simulink model "MSDR_and_BOP_v1_1"  (R2019a)
settings: Solver=ode45  StartTime=0.0  StopTime=15000  FixedStep=0.1  MaxStep=10
values from neighbouring files (symbols this model uses):
  a_f = -3.22E-5    (= -3.22e-05)    [MSDR_parameters_v1_1.m]
  a_g = +2.35E-5    (= 2.35e-05)    [MSDR_parameters_v1_1.m]
  A_s = 1.2245    [MSDR_parameters_v1_1.m]
  beta = [0.000223, 0.001457, 0.001307, 0.002628, 0.000766, 0.000280]    [MSDR_parameters_v1_1.m]
  beta_t = sum(beta)    [MSDR_parameters_v1_1.m]
  ce1 = 1.2471e-07    [MSDR_parameters_v1_1.m]
  ce2 = 5.3816e-14    [MSDR_parameters_v1_1.m]
  ce3 = 3.3721e-08    [MSDR_parameters_v1_1.m]
  Cp_fw = 3200.448e-6    (= 0.003200448)    [MSDR_parameters_v1_1.m]
  Cp_hr = 0.0021520    (= 0.002152)    [MSDR_parameters_v1_1.m]
  Cp_p = Cp_s_shx    (= 0.00154912)    [MSDR_parameters_v1_1.m]
  Cp_s = Cp_s*1e-6    (= 3.588208e-09)    [MSDR_parameters_v1_1.m]
  Cp_s_shx = 1549.12e-6    (= 0.00154912)    [MSDR_parameters_v1_1.m]
  Cp_sc = 4761.392e-6    (= 0.004761392)    [MSDR_parameters_v1_1.m]
  Cp_w = 456.056e-6    (= 0.000456056)    [MSDR_parameters_v1_1.m]
  D_it = 0.0141478    [MSDR_parameters_v1_1.m]
  D_ot = 0.015875    [MSDR_parameters_v1_1.m]
  dHs_dPs = -0.042433622114357    (= -0.0424336221144)    [MSDR_parameters_v1_1.m]
  eta_hp_isen = 0.861    [MSDR_parameters_v1_1.m]
  eta_lp_isen = 0.861    [MSDR_parameters_v1_1.m]
  gamma_I = 5.1135e-2    (= 0.051135)    [MSDR_parameters_v1_1.m]
  gamma_Xe = 1.1628e-2    (= 0.011628)    [MSDR_parameters_v1_1.m]
  H_fwh1 = 0.46009    [MSDR_parameters_v1_1.m]
  h_fwh1 = 0.5927    [MSDR_parameters_v1_1.m]
  H_fwh2 = 0.6784    [MSDR_parameters_v1_1.m]
  h_fwh2 = 0.5927    [MSDR_parameters_v1_1.m]
  H_lp_isen = 958.4*1054.35e-6/0.45359237    (= 2.22774699671)    [MSDR_parameters_v1_1.m]
  H_nc = 3.2952    [MSDR_parameters_v1_1.m]
  h_pw = h_s_shx    (= 0.00567446)    [MSDR_parameters_v1_1.m]
  H_rh = 2.8115    [MSDR_parameters_v1_1.m]
  h_wb = 13349.334646671E-6    (= 0.0133493346467)    [MSDR_parameters_v1_1.m]
  h_ws = 5732.378387768E-6    (= 0.00573237838777)    [MSDR_parameters_v1_1.m]
  h_wsc = 8385.005556375E-6    (= 0.00838500555638)    [MSDR_parameters_v1_1.m]
  hA_fg = [h_fg*A_fg/2, h_fg*A_fg/2]    [MSDR_parameters_v1_1.m]
  hA_p_phx1 = h_p_phx*A_p_phx    [MSDR_parameters_v1_1.m]
  hA_p_phx2 = h_p_phx*A_p_phx    [MSDR_parameters_v1_1.m]
  hA_p_phx3 = h_p_phx*A_p_phx    [MSDR_parameters_v1_1.m]
  hA_p_phx4 = h_p_phx*A_p_phx    [MSDR_parameters_v1_1.m]
  hA_p_phx5 = h_p_phx*A_p_phx    [MSDR_parameters_v1_1.m]
  hA_p_phx6 = h_p_phx*A_p_phx    [MSDR_parameters_v1_1.m]
  hA_p_shx1 = h_p_shx*A_p_shx    [MSDR_parameters_v1_1.m]
  hA_p_shx2 = h_p_shx*A_p_shx    [MSDR_parameters_v1_1.m]
  hA_p_shx3 = h_p_shx*A_p_shx    [MSDR_parameters_v1_1.m]
  hA_p_shx4 = h_p_shx*A_p_shx    [MSDR_parameters_v1_1.m]
  hA_p_shx5 = h_p_shx*A_p_shx    [MSDR_parameters_v1_1.m]
  hA_p_shx6 = h_p_shx*A_p_shx    [MSDR_parameters_v1_1.m]
  hA_s_phx1 = h_s_phx*A_s_phx    [MSDR_parameters_v1_1.m]
  hA_s_phx2 = h_s_phx*A_s_phx    [MSDR_parameters_v1_1.m]
  hA_s_phx3 = h_s_phx*A_s_phx    [MSDR_parameters_v1_1.m]
  hA_s_phx4 = h_s_phx*A_s_phx    [MSDR_parameters_v1_1.m]
  hA_s_phx5 = h_s_phx*A_s_phx    [MSDR_parameters_v1_1.m]
  hA_s_phx6 = h_s_phx*A_s_phx    [MSDR_parameters_v1_1.m]
  hA_s_shx1 = h_s_shx*A_s_shx    [MSDR_parameters_v1_1.m]
  hA_s_shx2 = h_s_shx*A_s_shx    [MSDR_parameters_v1_1.m]
  hA_s_shx3 = h_s_shx*A_s_shx    [MSDR_parameters_v1_1.m]
  hA_s_shx4 = h_s_shx*A_s_shx    [MSDR_parameters_v1_1.m]
  hA_s_shx5 = h_s_shx*A_s_shx    [MSDR_parameters_v1_1.m]
  hA_s_shx6 = h_s_shx*A_s_shx    [MSDR_parameters_v1_1.m]
  I_0 = gamma_I*Sig_f_msdr*phi_0/lam_I    (= 4.38204721773e+16)    [MSDR_parameters_v1_1.m]
  Ifa = [0.25, 0.25]    [MSDR_parameters_v1_1.m]
  Ifb = [0.25, 0.25]    [MSDR_parameters_v1_1.m]
  Ig = [0.5, 0.5]    [MSDR_parameters_v1_1.m]
  K_1 = 11.632248097704855    (= 11.6322480977)    [MSDR_parameters_v1_1.m]
  K_4 = b(1)    [MSDR_parameters_v1_1.m]
  K_5 = a(1)    [MSDR_parameters_v1_1.m]
  K_b = 12.834854076292217    (= 12.8348540763)    [MSDR_parameters_v1_1.m]
  K_b_hp = 0.1634    [MSDR_parameters_v1_1.m]
  K_b_lp = 0.2174    [MSDR_parameters_v1_1.m]
  K_sc = -17.615718797133468    (= -17.6157187971)    [MSDR_parameters_v1_1.m]
  ka = [0.235, 0.235]    [MSDR_parameters_v1_1.m]
  kb = [0.235, 0.235]    [MSDR_parameters_v1_1.m]
  kga = [0.015, 0.015]    [MSDR_parameters_v1_1.m]
  kgb = [0.015, 0.015]    [MSDR_parameters_v1_1.m]
  L = 8.5344    [MSDR_parameters_v1_1.m]
  L_b = 2.3645    [MSDR_parameters_v1_1.m]
  L_s = 4.723    [MSDR_parameters_v1_1.m]
  Lam = 2.400E-04    (= 0.00024)    [MSDR_parameters_v1_1.m]
  lam = [0.0124, 0.0305, 0.111, 0.301, 1.14, 3.01]    [MSDR_parameters_v1_1.m]
  lam_bubl = 2.0e-2    (= 0.02)    [MSDR_parameters_v1_1.m]
  lam_I = 2.875e-5    (= 2.875e-05)    [MSDR_parameters_v1_1.m]
  lam_Xe = 2.0916e-5    (= 2.0916e-05)    [MSDR_parameters_v1_1.m]
  m_3m = W_3*2    (= 8618.207327)    [MSDR_parameters_v1_1.m]
  m_fm = W_f*2    (= 9978.96)    [MSDR_parameters_v1_1.m]
  m_sb = 1717    [MSDR_parameters_v1_1.m]
  M_stm = 0.018    [MSDR_parameters_v1_1.m]
  mb_cpb = 2.689619410657651e+00    (= 2.68961941066)    [MSDR_parameters_v1_1.m]
  mcp_fa = mfa*Cp_f    [MSDR_parameters_v1_1.m]
  mcp_fb = mfb*Cp_f    [MSDR_parameters_v1_1.m]
  mcp_g = mg*Cp_g    [MSDR_parameters_v1_1.m]
  mcp_p_phx1 = Cp_p_phx*mp_phx1    [MSDR_parameters_v1_1.m]
  mcp_p_phx2 = Cp_p_phx*mp_phx2    [MSDR_parameters_v1_1.m]
  mcp_p_phx3 = Cp_p_phx*mp_phx3    [MSDR_parameters_v1_1.m]
  mcp_p_phx4 = Cp_p_phx*mp_phx4    [MSDR_parameters_v1_1.m]
  mcp_p_phx5 = Cp_p_phx*mp_phx5    [MSDR_parameters_v1_1.m]
  mcp_p_phx6 = Cp_p_phx*mp_phx6    [MSDR_parameters_v1_1.m]
  mcp_p_shx1 = Cp_p_shx*mp_shx1    [MSDR_parameters_v1_1.m]
  mcp_p_shx2 = Cp_p_shx*mp_shx2    [MSDR_parameters_v1_1.m]
  mcp_p_shx3 = Cp_p_shx*mp_shx3    [MSDR_parameters_v1_1.m]
  mcp_p_shx4 = Cp_p_shx*mp_shx4    [MSDR_parameters_v1_1.m]
  mcp_p_shx5 = Cp_p_shx*mp_shx5    [MSDR_parameters_v1_1.m]
  mcp_p_shx6 = Cp_p_shx*mp_shx6    [MSDR_parameters_v1_1.m]
  mcp_s_phx1 = Cp_s_phx*ms_phx1    [MSDR_parameters_v1_1.m]
  mcp_s_phx2 = Cp_s_phx*ms_phx2    [MSDR_parameters_v1_1.m]
  mcp_s_phx3 = Cp_s_phx*ms_phx3    [MSDR_parameters_v1_1.m]
  mcp_s_phx4 = Cp_s_phx*ms_phx4    [MSDR_parameters_v1_1.m]
  mcp_s_phx5 = Cp_s_phx*ms_phx5    [MSDR_parameters_v1_1.m]
  mcp_s_phx6 = Cp_s_phx*ms_phx6    [MSDR_parameters_v1_1.m]
  mcp_s_shx1 = Cp_s_shx*ms_shx1    [MSDR_parameters_v1_1.m]
  mcp_s_shx2 = Cp_s_shx*ms_shx1    [MSDR_parameters_v1_1.m]
  mcp_s_shx3 = Cp_s_shx*ms_shx1    [MSDR_parameters_v1_1.m]
  mcp_s_shx4 = Cp_s_shx*ms_shx1    [MSDR_parameters_v1_1.m]
  mcp_s_shx5 = Cp_s_shx*ms_shx1    [MSDR_parameters_v1_1.m]
  mcp_s_shx6 = Cp_s_shx*ms_shx1    [MSDR_parameters_v1_1.m]
  mcp_t_phx1 = Cp_t_phx*mt_phx1    [MSDR_parameters_v1_1.m]
  mcp_t_phx2 = Cp_t_phx*mt_phx2    [MSDR_parameters_v1_1.m]
  mcp_t_phx3 = Cp_t_phx*mt_phx3    [MSDR_parameters_v1_1.m]
  mcp_t_phx4 = Cp_t_phx*mt_phx4    [MSDR_parameters_v1_1.m]
  mcp_t_phx5 = Cp_t_phx*mt_phx5    [MSDR_parameters_v1_1.m]
  mcp_t_phx6 = Cp_t_phx*mt_phx6    [MSDR_parameters_v1_1.m]
  mcp_t_shx1 = Cp_t_phx*mt_shx1    [MSDR_parameters_v1_1.m]
  ... (+177 more)
undefined symbols (not defined in the file or in its folder): C0, H_con_table, H_convap_table, H_rh_table, H_rh_table1, H_rh_table2, H_rhvap_table, H_s_table, H_table, hA_p_thx1, hA_p_thx2, hA_p_thx3, hA_s_thx1, hA_s_thx2, hA_s_thx3, ln, mcp_p_thx1, mcp_p_thx2, mcp_p_thx3, mcp_s_thx1, mcp_s_thx2, mcp_s_thx3, mcp_t_thx1, mcp_t_thx2, mcp_t_thx3, mp_thx1, mp_thx2, mp_thx3, ms_thx1, ms_thx2, ms_thx3, P_con_table, P_nc_table, P_rh_table, P_rh_table1, pres_table, rho_rh_table, rho_table, SV_nc_table, T0_p_thx1, T0_p_thx2, T0_p_thx3, T0_s_thx1, T0_s_thx2, T0_s_thx3, T0_t_thx1, T0_t_thx2, T0_t_thx3, temp_table, u14, Wp_thx1, Wp_thx2, Wp_thx3, Ws_thx1, Ws_thx2, Ws_thx3
libraries: simulink x10
(part 2 of 4)

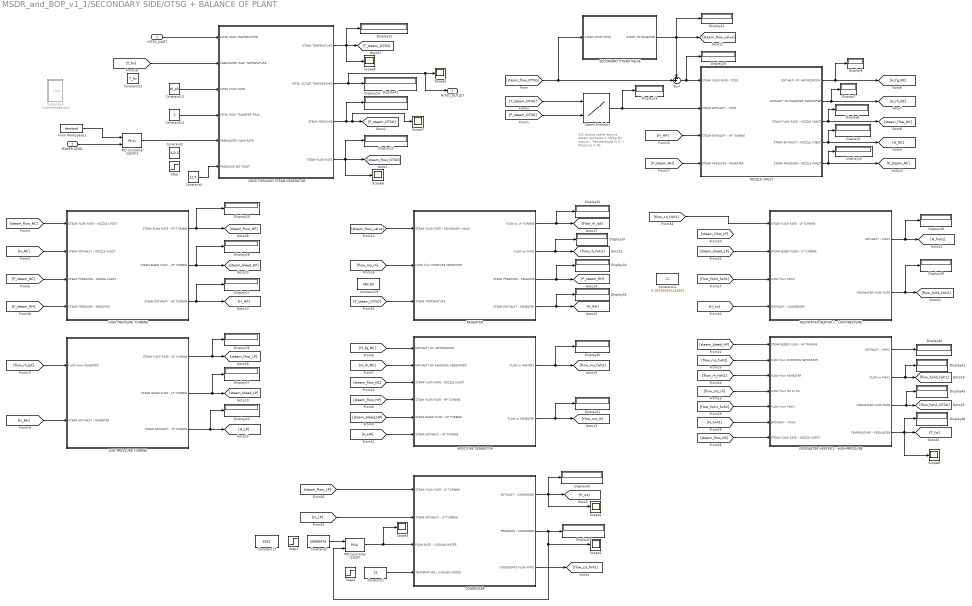
== system MSDR_and_BOP_v1_1/SECONDARY SIDE/OTSG + BALANCE OF PLANT ==
  note: 2-D lookup table returns steam enthalpy in MJ/kg for inputs i. Temperature in C, ii. Pressure in Pa
  HITEC_INLET : Inport
  POWER LEVEL : Inport  Port=2
  CONDENSER : Subsystem
  Constant1 : Constant  Value=15
  Constant11 : Constant  Value=0.160386626432892
  Constant12 : Constant  Value=T_fw
  Constant13 : Constant  Value=W_p0
  Constant14 : Constant
  Constant17 : Constant  Value=2552
  Constant19 : Constant  Value=482.63
  Constant2 : Constant  Value=322.5
  Constant3 : Constant  Value=.00689476
  Constant4 : Constant  Value=12.5
  Display{6..15,26..47} (32 alike) : Display
  FEEDWATER HEATER 1 - LOW-PRESSURE : Subsystem
  FEEDWATER HEATER 2 - HIGH-PRESSURE : Subsystem
  From Workspace1 : FromWorkspace  VariableName=demand  SampleTime=1  Interpolate=off  OutputAfterFinalValue=Holding final value
  HIGH PRESSURE TURBINE : Subsystem
  LOW PRESSURE TURBINE : Subsystem
  MOISTURE SEPARATOR : Subsystem
  NOZZLE CHEST : Subsystem
  ONCE-THROUGH STEAM GENERATOR : Subsystem
  PID Controller (2DOF) : simulink/Continuous/PID Controller (2DOF)  Controller=PI  Form=Ideal  TimeDomain=Continuous-time  SampleTime=-1  IntegratorMethod=Forward Euler  FilterMethod=Forward Euler  ControllerParametersSource=internal  P=-10020.0301151595  I=2.45363177832513  D=1  UseFilter=on  N=100  b=8.59224632013355e-05  c=1  TunerSelectOption=Transfer Function Based (PID Tuner App)  InitialConditionSource=internal  InitialConditionForIntegrator=0  InitialConditionForFilter=0  DifferentiatorICPrevScaledInput=0  ExternalReset=none  TrackingMode=off  Kt=1  LimitOutput=on  UpperSaturationLimit=100000  LowerSaturationLimit=10  LinearizeAsGain=off  AntiWindupMode=none  Kb=1  POutMin=[]  POutMax=[]  IOutMin=[]  IOutMax=[]  DOutMin=[]  DOutMax=[]  NOutMin=[]  NOutMax=[]  bOutMin=[]  bOutMax=[]  cOutMin=[]  cOutMax=[]  SumOutMin=[]  SumOutMax=[]  SaturationOutMin=[]  SaturationOutMax=[]  PParamMin=[]  PParamMax=[]  IParamMin=[]  IParamMax=[]  DParamMin=[]  DParamMax=[]  NParamMin=[]  NParamMax=[]  bParamMin=[]  bParamMax=[]  cParamMin=[]  cParamMax=[]  KbParamMin=[]  KbParamMax=[]  KtParamMin=[]  KtParamMax=[]  KbOutMin=[]  KbOutMax=[]  KtOutMin=[]  KtOutMax=[]  IntegratorOutMin=[]  IntegratorOutMax=[]  FilterOutMin=[]  FilterOutMax=[]  SumI1OutMin=[]  SumI1OutMax=[]  SumI2OutMin=[]  SumI2OutMax=[]  SumI3OutMin=[]  SumI3OutMax=[]  SumI4OutMin=[]  SumI4OutMax=[]  SumDOutMin=[]  SumDOutMax=[]  Sum1OutMin=[]  Sum1OutMax=[]  Sum2OutMin=[]  Sum2OutMax=[]  Sum3OutMin=[]  Sum3OutMax=[]  DifferentiatorOutMin=[]  DifferentiatorOutMax=[]  FilterDiffOutCoefMin=[]  FilterDiffOutCoefMax=[]  ReciprocalOutMin=[]  ReciprocalOutMax=[]  SumDenOutMin=[]  SumDenOutMax=[]  SumNumOutMin=[]  SumNumOutMax=[]  DivideOutMin=[]  DivideOutMax=[]  IntegratorContinuousStateAttributes=''  IntegratorStateMustResolveToSignalObject=off  IntegratorRTWStateStorageClass=Auto  FilterContinuousStateAttributes=''  FilterStateMustResolveToSignalObject=off  FilterRTWStateStorageClass=Auto  ParallelPVariant=Passthrough  IdealPVariant=InternalParameters  IVariant=InternalParameters  DVariant=Disabled  bVariant=InternalParameters  cVariant=Disabled  IntegratorVariant=Continuous  SatVariant=Enabled  AWVariant=Passthrough  PCopyVariant=Disabled  TRVariant=Disabled  FdbkBlocksVariant=Forward  IdealPFdbkVariant=Disabled  SatFdbkVariant=Disabled  DerivativeFilterVariant=Disabled  NVariant=Disabled  NCopyVariant=Disabled_SignalSpec  FilterICVariant=Disabled  IntegratorICVariant=InternalICs  ExternalResetVariant=Disabled  TRSumVariant=Passthrough  SumFdbkVariant=Disabled  SumVariant=Sum_PI
  PID Controller (2DOF)1 : simulink/Continuous/PID Controller (2DOF)  Controller=PI  Form=Parallel  TimeDomain=Continuous-time  SampleTime=-1  IntegratorMethod=Forward Euler  FilterMethod=Forward Euler  ControllerParametersSource=internal  P=250  I=5  D=1  UseFilter=on  N=100  b=1  c=1  TunerSelectOption=Transfer Function Based (PID Tuner App)  InitialConditionSource=internal  InitialConditionForIntegrator=0  InitialConditionForFilter=0  DifferentiatorICPrevScaledInput=0  ExternalReset=none  TrackingMode=off  Kt=1  LimitOutput=on  UpperSaturationLimit=1000000  LowerSaturationLimit=1  LinearizeAsGain=on  AntiWindupMode=none  Kb=1  POutMin=[]  POutMax=[]  IOutMin=[]  IOutMax=[]  DOutMin=[]  DOutMax=[]  NOutMin=[]  NOutMax=[]  bOutMin=[]  bOutMax=[]  cOutMin=[]  cOutMax=[]  SumOutMin=[]  SumOutMax=[]  SaturationOutMin=[]  SaturationOutMax=[]  PParamMin=[]  PParamMax=[]  IParamMin=[]  IParamMax=[]  DParamMin=[]  DParamMax=[]  NParamMin=[]  NParamMax=[]  bParamMin=[]  bParamMax=[]  cParamMin=[]  cParamMax=[]  KbParamMin=[]  KbParamMax=[]  KtParamMin=[]  KtParamMax=[]  KbOutMin=[]  KbOutMax=[]  KtOutMin=[]  KtOutMax=[]  IntegratorOutMin=[]  IntegratorOutMax=[]  FilterOutMin=[]  FilterOutMax=[]  SumI1OutMin=[]  SumI1OutMax=[]  SumI2OutMin=[]  SumI2OutMax=[]  SumI3OutMin=[]  SumI3OutMax=[]  SumI4OutMin=[]  SumI4OutMax=[]  SumDOutMin=[]  SumDOutMax=[]  Sum1OutMin=[]  Sum1OutMax=[]  Sum2OutMin=[]  Sum2OutMax=[]  Sum3OutMin=[]  Sum3OutMax=[]  DifferentiatorOutMin=[]  DifferentiatorOutMax=[]  FilterDiffOutCoefMin=[]  FilterDiffOutCoefMax=[]  ReciprocalOutMin=[]  ReciprocalOutMax=[]  SumDenOutMin=[]  SumDenOutMax=[]  SumNumOutMin=[]  SumNumOutMax=[]  DivideOutMin=[]  DivideOutMax=[]  IntegratorContinuousStateAttributes=''  IntegratorStateMustResolveToSignalObject=off  IntegratorRTWStateStorageClass=Auto  FilterContinuousStateAttributes=''  FilterStateMustResolveToSignalObject=off  FilterRTWStateStorageClass=Auto  ParallelPVariant=InternalParameters  IdealPVariant=Disabled  IVariant=InternalParameters  DVariant=Disabled  bVariant=InternalParameters  cVariant=Disabled  IntegratorVariant=Continuous  SatVariant=Enabled  AWVariant=Passthrough  PCopyVariant=Disabled  TRVariant=Disabled  FdbkBlocksVariant=Forward  IdealPFdbkVariant=Disabled  SatFdbkVariant=Disabled  DerivativeFilterVariant=Disabled  NVariant=Disabled  NCopyVariant=Disabled_SignalSpec  FilterICVariant=Disabled  IntegratorICVariant=InternalICs  ExternalResetVariant=Disabled  TRSumVariant=Passthrough  SumFdbkVariant=Disabled  SumVariant=Sum_PI
  REHEATER : Subsystem
  SECONDARY STEAM VALVE : Subsystem
  Scope{1..8} (8 alike) : Scope
  Steam Enthalpy : Lookup_n-D  BreakpointsForDimension1=temp_table  BreakpointsForDimension2=pres_table  Table=H_s_table  DiagnosticForOutOfRangeInput=Warning  InternalRulePriority=Speed  RndMeth=Simplest  InputSameDT=on
  Step : Step  Time=1000  Before=12.5  After=12  SampleTime=0
  Step1 : Step  Time=1000  Before=0.00689476  After=.00589476  SampleTime=0
  Step2 : Step  Time=1000  Before=25  After=15  SampleTime=0
  Subsystem : Subsystem  Commented=on
  Sum : Sum  Inputs=-+|
  HITEC_OUTLET : Outport
  wires:
  REHEATER/1("FLOW to LP TURBINE ") -> [flow_rh_lpt], Display32/1
  [steam_flow_NC] -> HIGH PRESSURE TURBINE/1(STEAM FLOW RATE - NOZZLE CHEST)
  [steam_bleed_HP] -> MOISTURE SEPARATOR/5(STEAM BLEED FLOW - HP TURBINE)
  [steam_flow_NC] -> MOISTURE SEPARATOR/3(STEAM FLOW RATE - NOZZLE CHEST)
  NOZZLE CHEST/3(STEAM FLOW RATE - NOZZLE CHEST) -> [steam_flow_NC], Display8/1
  [H_rh_NC] -> MOISTURE SEPARATOR/2(ENTHALPY OF REHEATER FEEDWATER)
  NOZZLE CHEST/2(ENTHALPY OF REHEATER FEEDWATER) -> [H_rh_NC], Display7/1
  [H_NC] -> HIGH PRESSURE TURBINE/2(STEAM ENTHALPY - NOZZLE CHEST)
  Steam Enthalpy/1 -> NOZZLE CHEST/2(STEAM ENTHALPY - OTSG), Display13/1
  [steam_flow_HP] -> MOISTURE SEPARATOR/4(STEAM FLOW RATE - HP TURBINE)
  Sum/1 -> Display26/1, NOZZLE CHEST/1(STEAM FLOW RATE - OTSG)
  NOZZLE CHEST/5(STEAM PRESSURE - NOZZLE CHEST) -> [P_steam_NC], Display10/1
  [H_fwh1] -> FEEDWATER HEATER 2 - HIGH-PRESSURE/6(ENTHALPY - FWH1)
  REHEATER/2(FLOW to FWH2) -> [flow_rh_fwh2], Display33/1
  FEEDWATER HEATER 1 - LOW-PRESSURE/1(ENTHALPY - FWH1) -> [H_fwh1], Display38/1
  [flow_rh_fwh2] -> FEEDWATER HEATER 2 - HIGH-PRESSURE/3(FLOW from REHEATER)
  [flow_ms_rh] -> FEEDWATER HEATER 2 - HIGH-PRESSURE/4(FLOW from MS to RH)
  FEEDWATER HEATER 2 - HIGH-PRESSURE/2(FLOW to FWH1) -> Display41/1, [flow_fwh2_fwh1]
  [flow_ms_fwh2] -> FEEDWATER HEATER 2 - HIGH-PRESSURE/2(FLOW from MOISTURE SEPARATOR)
  MOISTURE SEPARATOR/1(FLOW to HEATER2) -> [flow_ms_fwh2], Display30/1
  [flow_fwh2_fwh1] -> FEEDWATER HEATER 1 - LOW-PRESSURE/3(FLOW from FWH2)
  [flow_ms_rh] -> REHEATER/2(FLOW from MOISTURE SEPARATOR)
  MOISTURE SEPARATOR/2(FLOW to REHEATER) -> [flow_ms_rh], Display31/1
  REHEATER/3(STEAM PRESSURE - REHEATER) -> [P_steam_RH], Display34/1
  FEEDWATER HEATER 2 - HIGH-PRESSURE/3(FEEDWATER FLOW RATE) -> Display45/1, [flow_fwh2_OTSG]
  LOW PRESSURE TURBINE/3(STEAM ENTHALPY - LP TURBINE) -> Display42/1, [H_LP]
  [P_steam_NC] -> HIGH PRESSURE TURBINE/3(STEAM PRESSURE - NOZZLE CHEST)
  FEEDWATER HEATER 2 - HIGH-PRESSURE/4(TEMPERATURE - FEEDWATER) -> [T_fw], Scope8/1, Display46/1
  NOZZLE CHEST/4(STEAM ENTHALPY - NOZZLE CHEST) -> [H_NC], Display9/1
  [flow_rh_lpt] -> LOW PRESSURE TURBINE/1(FLOW from REHEATER)
  HIGH PRESSURE TURBINE/3(STEAM ENTHALPY - HP TURBINE) -> [H_HP], Display27/1
  [H_fg_NC] -> MOISTURE SEPARATOR/1(ENTHALPY OF VAPORIZATION)
  [flow_fwh1_fwh2] -> FEEDWATER HEATER 2 - HIGH-PRESSURE/5(FLOW from FWH1)
  [steam_flow_valve] -> REHEATER/1(STEAM FLOW RATE - SECONDARY VALVE)
  ONCE-THROUGH STEAM GENERATOR/4(STEAM FLOW RATE) -> Scope6/1, [steam_flow_OTSG], Display15/1
  [P_steam_OTSG] -> Steam Enthalpy/2
  [H_HP] -> MOISTURE SEPARATOR/6(STEAM ENTHALPY - HP TURBINE)
  SECONDARY STEAM VALVE/1(STEAM TO REHEATER) -> Display11/1, [steam_flow_valve], Sum/1
  [H_HP] -> NOZZLE CHEST/3(STEAM ENTHALPY - HP TURBINE)
  ONCE-THROUGH STEAM GENERATOR/2(HITEC OUTLET TEMPERATURE) -> HITEC_OUTLET/1, Scope5/1, Display47/1
  NOZZLE CHEST/1(ENTHALPY OF VAPORIZATION) -> [H_fg_NC], Display6/1
  [P_steam_RH] -> NOZZLE CHEST/4(STEAM PRESSURE - REHEATER)
  REHEATER/4(STEAM ENTHALPY - REHEATER) -> [H_RH], Display35/1
  LOW PRESSURE TURBINE/2(STEAM BLEED FLOW - LP TURBINE) -> [steam_bleed_LP], Display37/1
  Constant13/1 -> ONCE-THROUGH STEAM GENERATOR/3(HITEC FLOW RATE)
  FEEDWATER HEATER 2 - HIGH-PRESSURE/1(ENTHALPY - FWH2) -> Display40/1
  HIGH PRESSURE TURBINE/1(STEAM FLOW RATE - HP TURBINE) -> [steam_flow_HP], Display29/1
  [T_steam_OTSG] -> REHEATER/3(STEAM TEMPERATURE)
  ONCE-THROUGH STEAM GENERATOR/1(STEAM TEMPERATURE) -> Scope4/1, Display12/1, [T_steam_OTSG]
  Constant14/1 -> ONCE-THROUGH STEAM GENERATOR/4(HITEC HEAT TRANSFER FRAC)
  [T_fw] -> ONCE-THROUGH STEAM GENERATOR/2(FEEDWATER INLET TEMPERATURE)
  [steam_bleed_LP] -> FEEDWATER HEATER 1 - LOW-PRESSURE/2(STEAM BLEED FLOW - LP TURBINE)
  [H_RH] -> LOW PRESSURE TURBINE/2(STEAM ENTHALPY - REHEATER)
  [steam_bleed_HP] -> FEEDWATER HEATER 2 - HIGH-PRESSURE/1(STEAM BLEED FLOW - HP TURBINE)
  ONCE-THROUGH STEAM GENERATOR/3(STEAM PRESSURE) -> Scope7/1, [P_steam_OTSG], Display14/1
  LOW PRESSURE TURBINE/1(STEAM FLOW RATE - LP TURBINE) -> [steam_flow_LP], Display36/1
  [T_steam_OTSG] -> Steam Enthalpy/1
  [P_steam_RH] -> HIGH PRESSURE TURBINE/4(STEAM PRESSURE - REHEATER)
  HIGH PRESSURE TURBINE/2(STEAM BLEED FLOW - HP TURBINE) -> [steam_bleed_HP], Display28/1
  [steam_flow_NC] -> FEEDWATER HEATER 2 - HIGH-PRESSURE/7(STEAM FLOW RATE - NOZZLE CHEST)
  FEEDWATER HEATER 1 - LOW-PRESSURE/2(FEEDWATER FLOW RATE) -> Display39/1, [flow_fwh1_fwh2]
  [steam_flow_OTSG] -> SECONDARY STEAM VALVE/1(STEAM FROM OTSG), Sum/2
  HITEC_INLET/1 -> ONCE-THROUGH STEAM GENERATOR/1(HITEC INLET TEMPERATURE)
  POWER LEVEL/1 -> PID Controller (2DOF)1/2
  PID Controller (2DOF)/1 -> CONDENSER/3(FLOW RATE - COOLING WATER), Scope3/1
  CONDENSER/2(PRESSURE - CONDENSER) -> PID Controller (2DOF)/2, Scope1/1, Display44/1
  CONDENSER/1(ENTHALPY - CONDENSER) -> Scope2/1, [H_co], Display43/1
  [H_LP] -> CONDENSER/2(STEAM ENTHALPY - LP TURBINE)
  [steam_flow_LP] -> CONDENSER/1(STEAM FLOW RATE - LP TURBINE)
  [H_co] -> FEEDWATER HEATER 1 - LOW-PRESSURE/4(ENTHALPY - CONDENSER)
  CONDENSER/3(CONDENSATE FLOW RATE) -> [flow_co_fwh1]
  [flow_co_fwh1] -> FEEDWATER HEATER 1 - LOW-PRESSURE/1(STEAM FLOW RATE - LP TURBINE)
  From Workspace1/1 -> PID Controller (2DOF)1/1
  Constant3/1 -> PID Controller (2DOF)/1
  Constant1/1 -> CONDENSER/4(TEMPERATURE - COOLING WATER)
  Constant4/1 -> ONCE-THROUGH STEAM GENERATOR/6(PRESSURE SET POINT)
  PID Controller (2DOF)1/1 -> ONCE-THROUGH STEAM GENERATOR/5(FEEDWATER FLOW RATE)

== system MSDR_and_BOP_v1_1/HEAT EXCHANGERS/HEAT EXCHANGER LOOP 4/BOILER & REHEATER ==
  Coolant Inlet Temp : Inport
  Power Demand (Frac) : Inport  Port=2
  Fcn : Fcn  Commented=on  Expr=u[1] - u[2]*250/((Ws_shx1 + Ws_shx2)*Cp_s_shx)
  Integrator : Integrator  InitialCondition=400
  Mux : Mux  Inputs=3
      settings: DisplayOption=signals
  To Workspace : ToWorkspace  VariableName=msdr_br_mux1  SampleTime=-1
  ddt_t_b = 1/tau_b*(t_bin-t_b)-p_b/mb_cpb : Fcn  Expr=W_sb*(u(1)-u(3))/m_sb - u(2)/mb_cpb
  Coolant Exit Temp : Outport
  wires:
  Mux/1 -> ddt_t_b = 1/tau_b*(t_bin-t_b)-p_b/mb_cpb/1, To Workspace/1
  Power Demand (Frac)/1 -> Mux/2
  Coolant Inlet Temp/1 -> Mux/1
  ddt_t_b = 1/tau_b*(t_bin-t_b)-p_b/mb_cpb/1 -> Integrator/1
  Integrator/1 -> Coolant Exit Temp/1, Mux/3

== system MSDR_and_BOP_v1_1/HEAT EXCHANGERS/HEAT EXCHANGER LOOP 4/Fractional Power Demand (fractional) ==
  Add : Sum
  Constant : Constant
  Saturation : Saturate  UpperLimit=1  LowerLimit=0.2
  Saturation1 : Saturate  UpperLimit=.8  LowerLimit=0
  Slider : SliderBlock
  down 1%/min : simulink/Sources/Ramp  slope=-0.01/60  start=2500  InitialOutput=1
  up 1%/min1 : simulink/Sources/Ramp  slope=0.01/60  start=2500+3600+5000  InitialOutput=0
  Power Demand(frac) : Outport
  wires:
  down 1%/min/1 -> Saturation/1
  Saturation/1 -> Add/1
  up 1%/min1/1 -> Saturation1/1
  Saturation1/1 -> Add/2
  Constant/1 -> Power Demand(frac)/1

== system MSDR_and_BOP_v1_1/HEAT EXCHANGERS/HEAT EXCHANGER LOOP 4/PHX PRIM MIXING ==
  Tp_phx1 : Inport
  Tp_phx2 : Inport  Port=2
  p_flow_frac : Inport  Port=3
  Fcn : Fcn  Expr=u[3]*Wp_phx1/mp_phxm*(u[1]-u[4]) + u[3]*Wp_phx2/mp_phxm*(u[2]-u[4])
  Integrator : Integrator  InitialCondition=Tf_in
  Mux : Mux
  Tp_phx_mix : Outport
  wires:
  Tp_phx1/1 -> Mux/1
  Tp_phx2/1 -> Mux/2
  Mux/1 -> Fcn/1
  p_flow_frac/1 -> Mux/3
  Fcn/1 -> Integrator/1
  Integrator/1 -> Tp_phx_mix/1, Mux/4

== system MSDR_and_BOP_v1_1/HEAT EXCHANGERS/HEAT EXCHANGER LOOP 4/PHX SEC MIXING ==
  Ts_phx1 : Inport
  Ts_phx2 : Inport  Port=2
  s_flow_frac : Inport  Port=3
  Fcn : Fcn  Expr=u[3]*Ws_phx1/ms_phxm*(u[1]-u[4]) + u[3]*Ws_phx2/ms_phxm*(u[2]-u[4])
  Integrator : Integrator  InitialCondition=T0_s_phx1(4)
  Mux : Mux
  Ts_phx_mix : Outport
  wires:
  Ts_phx1/1 -> Mux/1
  Ts_phx2/1 -> Mux/2
  Mux/1 -> Fcn/1
  s_flow_frac/1 -> Mux/3
  Fcn/1 -> Integrator/1
  Integrator/1 -> Ts_phx_mix/1, Mux/4

== system MSDR_and_BOP_v1_1/HEAT EXCHANGERS/HEAT EXCHANGER LOOP 4/PHX//SHX PUMP ==
  1-D Lookup Table : Lookup_n-D  NumberOfTableDimensions=1  BreakpointsForDimension1=xdat  Table=ydat  InternalRulePriority=Speed  RndMeth=Simplest  InputSameDT=on
  Clock : Clock
  Fcn : Fcn  Expr=exp((1/tau_p)*u)
  Final convection flow rate : Constant  Value=therm_conv
  Scope : Scope
  Subtract : Sum  Inputs=-+
  Switch : Switch  Criteria=u2 > Threshold
  Transport Delay : TransportDelay  DelayTime=300000000  InitialOutput=1
  FLOW FRACTION : Outport
  HEAT TRANSFER FRACTION : Outport  Port=2
  wires:
  Transport Delay/1 -> 1-D Lookup Table/1, Scope/1, FLOW FRACTION/1
  Clock/1 -> Fcn/1
  Switch/1 -> Transport Delay/1
  Fcn/1 -> Subtract/1, Switch/1
  Final convection flow rate/1 -> Subtract/2, Switch/3
  Subtract/1 -> Switch/2
  1-D Lookup Table/1 -> HEAT TRANSFER FRACTION/1

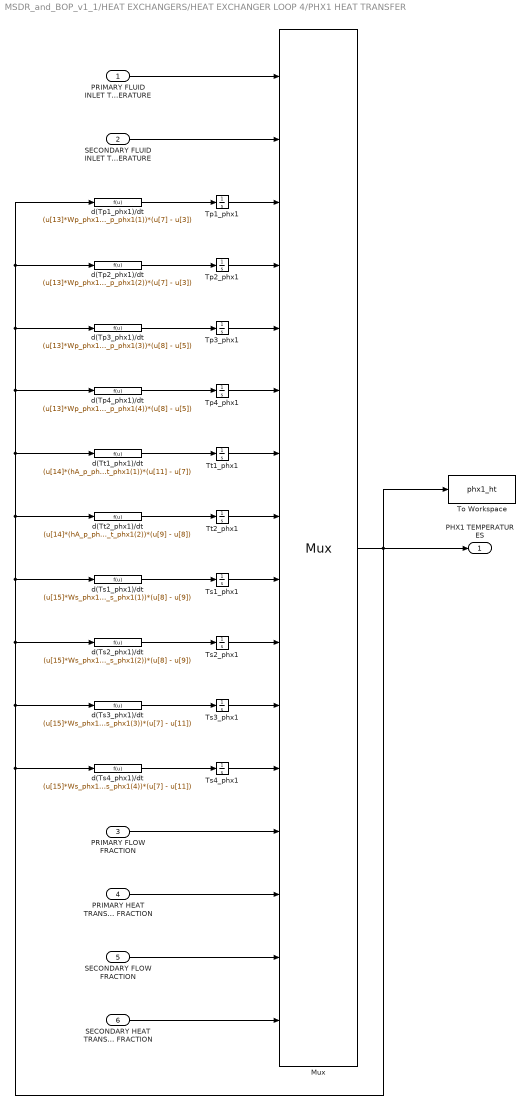
== system MSDR_and_BOP_v1_1/HEAT EXCHANGERS/HEAT EXCHANGER LOOP 4/PHX1 HEAT TRANSFER ==
  PRIMARY FLUID INLET TEMPERATURE : Inport
  SECONDARY FLUID INLET TEMPERATURE : Inport  Port=2
  PRIMARY FLOW FRACTION : Inport  Port=3
  PRIMARY HEAT TRANSFER FRACTION : Inport  Port=4
  SECONDARY FLOW FRACTION : Inport  Port=5
  SECONDARY HEAT TRANSFER FRACTION : Inport  Port=6
  Mux : Mux  Inputs=16
      settings: DisplayOption=signals
  To Workspace : ToWorkspace  VariableName=phx1_ht  SampleTime=-1
  Tp1_phx1 : Integrator  InitialCondition=T0_p_phx1(1)
  Tp2_phx1 : Integrator  InitialCondition=T0_p_phx1(2)
  "Tp3_phx1 " : Integrator  InitialCondition=T0_p_phx1(3)
  Tp4_phx1 : Integrator  InitialCondition=T0_p_phx1(4)
  Ts1_phx1 : Integrator  InitialCondition=T0_s_phx1(1)
  Ts2_phx1 : Integrator  InitialCondition=T0_s_phx1(2)
  Ts3_phx1 : Integrator  InitialCondition=T0_s_phx1(3)
  Ts4_phx1 : Integrator  InitialCondition=T0_s_phx1(4)
  Tt1_phx1 : Integrator  InitialCondition=T0_t_phx1(1)
  Tt2_phx1 : Integrator  InitialCondition=T0_t_phx1(2)
  d(Tp1_phx1)/dt : Fcn  Expr=(u[13]*Wp_phx1/mp_phx1(1))*(u[1] - u[3]) + (u[14]*hA_p_phx1(1)/mcp_p_phx1(1))*(u[7] - u[3])
  d(Tp2_phx1)/dt : Fcn  Expr=(u[13]*Wp_phx1/mp_phx1(2))*(u[3] - u[4]) + (u[14]*hA_p_phx1(2)/mcp_p_phx1(2))*(u[7] - u[3])
  d(Tp3_phx1)/dt : Fcn  Expr=(u[13]*Wp_phx1/mp_phx1(3))*(u[4] - u[5]) + (u[14]*hA_p_phx1(3)/mcp_p_phx1(3))*(u[8] - u[5])
  d(Tp4_phx1)/dt : Fcn  Expr=(u[13]*Wp_phx1/mp_phx1(4))*(u[5] - u[6]) + (u[14]*hA_p_phx1(4)/mcp_p_phx1(4))*(u[8] - u[5])
  d(Ts1_phx1)/dt : Fcn  Expr=(u[15]*Ws_phx1/ms_phx1(1))*(u[2] - u[9]) + (u[16]*hA_s_phx1(1)/mcp_s_phx1(1))*(u[8] - u[9])
  d(Ts2_phx1)/dt : Fcn  Expr=(u[15]*Ws_phx1/ms_phx1(2))*(u[9] - u[10]) + (u[16]*hA_s_phx1(2)/mcp_s_phx1(2))*(u[8] - u[9])
  d(Ts3_phx1)/dt : Fcn  Expr=(u[15]*Ws_phx1/ms_phx1(3))*(u[10] - u[11]) + (u[16]*hA_s_phx1(3)/mcp_s_phx1(3))*(u[7] - u[11])
  d(Ts4_phx1)/dt : Fcn  Expr=(u[15]*Ws_phx1/ms_phx1(4))*(u[11] - u[12]) + (u[16]*hA_s_phx1(4)/mcp_s_phx1(4))*(u[7] - u[11])
  d(Tt1_phx1)/dt : Fcn  Expr=(u[14]*(hA_p_phx1(1) + hA_p_phx1(2))/mcp_t_phx1(1))*(u[3] - u[7]) + (u[16]*(hA_s_phx1(1) + hA_s_phx1(2))/mcp_t_phx1(1))*(u[11] - u[7])
  d(Tt2_phx1)/dt : Fcn  Expr=(u[14]*(hA_p_phx1(3) + hA_p_phx1(4))/mcp_t_phx1(2))*(u[5] - u[8]) + (u[16]*(hA_s_phx1(3) + hA_s_phx1(4))/mcp_t_phx1(2))*(u[9] - u[8])
  PHX1 TEMPERATURES : Outport
  wires:
  Ts1_phx1/1 -> Mux/9
  Ts2_phx1/1 -> Mux/10
  d(Ts2_phx1)/dt/1 -> Ts2_phx1/1
  d(Tp4_phx1)/dt/1 -> Tp4_phx1/1
  Tt1_phx1/1 -> Mux/7
  d(Tp2_phx1)/dt/1 -> Tp2_phx1/1
  Tp4_phx1/1 -> Mux/6
  d(Tt2_phx1)/dt/1 -> Tt2_phx1/1
  SECONDARY FLUID INLET TEMPERATURE/1 -> Mux/2
  Tt2_phx1/1 -> Mux/8
  Mux/1 -> PHX1 TEMPERATURES/1, To Workspace/1, d(Ts4_phx1)/dt/1, d(Ts3_phx1)/dt/1, d(Ts1_phx1)/dt/1, d(Tt2_phx1)/dt/1, d(Tt1_phx1)/dt/1, d(Tp4_phx1)/dt/1, d(Tp3_phx1)/dt/1, d(Tp2_phx1)/dt/1, d(Tp1_phx1)/dt/1, d(Ts2_phx1)/dt/1
  d(Tp1_phx1)/dt/1 -> Tp1_phx1/1
  d(Ts4_phx1)/dt/1 -> Ts4_phx1/1
  Tp1_phx1/1 -> Mux/3
  d(Ts1_phx1)/dt/1 -> Ts1_phx1/1
  d(Ts3_phx1)/dt/1 -> Ts3_phx1/1
  Ts3_phx1/1 -> Mux/11
  Ts4_phx1/1 -> Mux/12
  "Tp3_phx1 "/1 -> Mux/5
  d(Tp3_phx1)/dt/1 -> "Tp3_phx1 "/1
  Tp2_phx1/1 -> Mux/4
  d(Tt1_phx1)/dt/1 -> Tt1_phx1/1
  PRIMARY FLUID INLET TEMPERATURE/1 -> Mux/1
  PRIMARY FLOW FRACTION/1 -> Mux/13
  PRIMARY HEAT TRANSFER FRACTION/1 -> Mux/14
  SECONDARY HEAT TRANSFER FRACTION/1 -> Mux/16
  SECONDARY FLOW FRACTION/1 -> Mux/15

== system MSDR_and_BOP_v1_1/HEAT EXCHANGERS/HEAT EXCHANGER LOOP 4/PHX1 MATERIAL TRANSPORT ==
  PHX1 TEMPERATURES : Inport
  wires:
  PHX1 TEMPERATURES/1 -> ?

== system MSDR_and_BOP_v1_1/HEAT EXCHANGERS/HEAT EXCHANGER LOOP 4/PHX2 HEAT TRANSFER ==
  PRIMARY FLUID INLET TEMPERATURE : Inport
  SECONDARY FLUID INLET TEMPERATURE : Inport  Port=2
  PRIMARY FLOW FRACTION : Inport  Port=3
  PRIMARY HEAT TRANSFER FRACTION : Inport  Port=4
  SECONDARY FLOW FRACTION : Inport  Port=5
  SECONDARY HEAT TRANSFER FRACTION : Inport  Port=6
  Mux : Mux  Inputs=16
      settings: DisplayOption=signals
  To Workspace : ToWorkspace  VariableName=phx2_ht  SampleTime=-1
  Tp1_phx2 : Integrator  InitialCondition=T0_p_phx2(1)
  Tp2_phx2 : Integrator  InitialCondition=T0_p_phx1(2)
  "Tp3_phx2 " : Integrator  InitialCondition=T0_p_phx2(3)
  Tp4_phx2 : Integrator  InitialCondition=T0_p_phx2(4)
  Ts1_phx2 : Integrator  InitialCondition=T0_s_phx2(1)
  Ts2_phx2 : Integrator  InitialCondition=T0_s_phx2(2)
  Ts3_phx2 : Integrator  InitialCondition=T0_s_phx2(3)
  Ts4_phx2 : Integrator  InitialCondition=T0_s_phx2(4)
  Tt1_phx2 : Integrator  InitialCondition=T0_t_phx2(1)
  Tt2_phx2 : Integrator  InitialCondition=T0_t_phx2(2)
  d(Tp1_phx2)/dt : Fcn  Expr=(u[13]*Wp_phx2/mp_phx2(1))*(u[1] - u[3]) + (u[14]*hA_p_phx2(1)/mcp_p_phx2(1))*(u[7] - u[3])
  d(Tp2_phx2)/dt : Fcn  Expr=(u[13]*Wp_phx2/mp_phx2(2))*(u[3] - u[4]) + (u[14]*hA_p_phx2(2)/mcp_p_phx2(2))*(u[7] - u[3])
  d(Tp3_phx2)/dt : Fcn  Expr=(u[13]*Wp_phx2/mp_phx2(3))*(u[4] - u[5]) + (u[14]*hA_p_phx2(3)/mcp_p_phx2(3))*(u[8] - u[5])
  d(Tp4_phx2)/dt : Fcn  Expr=(u[13]*Wp_phx2/mp_phx2(4))*(u[5] - u[6]) + (u[14]*hA_p_phx2(4)/mcp_p_phx2(4))*(u[8] - u[5])
  d(Ts1_phx2)/dt : Fcn  Expr=(u[15]*Ws_phx2/ms_phx2(1))*(u[2] - u[9]) + (u[16]*hA_s_phx2(1)/mcp_s_phx2(1))*(u[8] - u[9])
  d(Ts2_phx2)/dt : Fcn  Expr=(u[15]*Ws_phx2/ms_phx2(2))*(u[9] - u[10]) + (u[16]*hA_s_phx2(2)/mcp_s_phx2(2))*(u[8] - u[9])
  d(Ts3_phx2)/dt : Fcn  Expr=(u[15]*Ws_phx2/ms_phx2(3))*(u[10] - u[11]) + (u[16]*hA_s_phx2(3)/mcp_s_phx2(3))*(u[7] - u[11])
  d(Ts4_phx2)/dt : Fcn  Expr=(u[15]*Ws_phx2/ms_phx2(4))*(u[11] - u[12]) + (u[16]*hA_s_phx2(4)/mcp_s_phx2(4))*(u[7] - u[11])
  d(Tt1_phx2)/dt : Fcn  Expr=(u[14]*(hA_p_phx2(1) + hA_p_phx2(2))/mcp_t_phx2(1))*(u[3] - u[7]) + (u[16]*(hA_s_phx2(1) + hA_s_phx2(2))/mcp_t_phx2(1))*(u[11] - u[7])
  d(Tt2_phx2)/dt : Fcn  Expr=(u[14]*(hA_p_phx2(3) + hA_p_phx2(4))/mcp_t_phx2(2))*(u[5] - u[8]) + (u[16]*(hA_s_phx2(3) + hA_s_phx2(4))/mcp_t_phx2(2))*(u[9] - u[8])
  PHX2 TEMPERATURES : Outport
  wires:
  Ts1_phx2/1 -> Mux/9
  Ts2_phx2/1 -> Mux/10
  d(Ts2_phx2)/dt/1 -> Ts2_phx2/1
  d(Tp4_phx2)/dt/1 -> Tp4_phx2/1
  Tt1_phx2/1 -> Mux/7
  d(Tp2_phx2)/dt/1 -> Tp2_phx2/1
  Tp4_phx2/1 -> Mux/6
  d(Tt2_phx2)/dt/1 -> Tt2_phx2/1
  SECONDARY FLUID INLET TEMPERATURE/1 -> Mux/2
  Tt2_phx2/1 -> Mux/8
  Mux/1 -> To Workspace/1, PHX2 TEMPERATURES/1, d(Ts4_phx2)/dt/1, d(Ts3_phx2)/dt/1, d(Ts1_phx2)/dt/1, d(Tt2_phx2)/dt/1, d(Tt1_phx2)/dt/1, d(Tp4_phx2)/dt/1, d(Tp3_phx2)/dt/1, d(Tp2_phx2)/dt/1, d(Tp1_phx2)/dt/1, d(Ts2_phx2)/dt/1
  d(Tp1_phx2)/dt/1 -> Tp1_phx2/1
  d(Ts4_phx2)/dt/1 -> Ts4_phx2/1
  Tp1_phx2/1 -> Mux/3
  d(Ts1_phx2)/dt/1 -> Ts1_phx2/1
  d(Ts3_phx2)/dt/1 -> Ts3_phx2/1
  Ts3_phx2/1 -> Mux/11
  Ts4_phx2/1 -> Mux/12
  "Tp3_phx2 "/1 -> Mux/5
  d(Tp3_phx2)/dt/1 -> "Tp3_phx2 "/1
  Tp2_phx2/1 -> Mux/4
  d(Tt1_phx2)/dt/1 -> Tt1_phx2/1
  PRIMARY FLUID INLET TEMPERATURE/1 -> Mux/1
  PRIMARY FLOW FRACTION/1 -> Mux/13
  PRIMARY HEAT TRANSFER FRACTION/1 -> Mux/14
  SECONDARY FLOW FRACTION/1 -> Mux/15
  SECONDARY HEAT TRANSFER FRACTION/1 -> Mux/16

== system MSDR_and_BOP_v1_1/HEAT EXCHANGERS/HEAT EXCHANGER LOOP 4/PHX2 MATERIAL TRANSPORT ==
  PHX2 TEMPERATURES : Inport
  wires:
  PHX2 TEMPERATURES/1 -> ?

== system MSDR_and_BOP_v1_1/HEAT EXCHANGERS/HEAT EXCHANGER LOOP 4/SHX PRIM MIXING ==
  Tp_shx1 : Inport
  Tp_shx2 : Inport  Port=2
  p_flow_frac : Inport  Port=3
  Fcn : Fcn  Expr=u[3]*Wp_shx1/mp_shxm*(u[1]-u[4]) + u[3]*Wp_shx2/mp_shxm*(u[2]-u[4])
  Integrator : Integrator  InitialCondition=T0_p_shx1(4)
  Mux : Mux
  Tp_shx_mix : Outport
  wires:
  Tp_shx1/1 -> Mux/1
  Tp_shx2/1 -> Mux/2
  Mux/1 -> Fcn/1
  p_flow_frac/1 -> Mux/3
  Fcn/1 -> Integrator/1
  Integrator/1 -> Tp_shx_mix/1, Mux/4

== system MSDR_and_BOP_v1_1/HEAT EXCHANGERS/HEAT EXCHANGER LOOP 4/SHX SEC MIXING ==
  Ts_shx1 : Inport
  Ts_shx2 : Inport  Port=2
  s_flow_frac : Inport  Port=3
  Fcn : Fcn  Expr=u[3]*Ws_shx1/ms_shxm*(u[1]-u[4]) + u[3]*Ws_shx2/ms_shxm*(u[2]-u[4])
  Integrator : Integrator  InitialCondition=T0_s_shx1(4)
  Mux : Mux
  Ts_shx_mix : Outport
  wires:
  Ts_shx1/1 -> Mux/1
  Ts_shx2/1 -> Mux/2
  Mux/1 -> Fcn/1
  s_flow_frac/1 -> Mux/3
  Fcn/1 -> Integrator/1
  Integrator/1 -> Ts_shx_mix/1, Mux/4

== system MSDR_and_BOP_v1_1/HEAT EXCHANGERS/HEAT EXCHANGER LOOP 4/SHX//THX PUMP ==
  1-D Lookup Table : Lookup_n-D  NumberOfTableDimensions=1  BreakpointsForDimension1=xdat  Table=ydat  InternalRulePriority=Speed  RndMeth=Simplest  InputSameDT=on
  Clock : Clock
  Fcn : Fcn  Expr=exp((1/tau_p)*u)
  Final convection flow rate : Constant  Value=therm_conv
  Scope : Scope
  Subtract : Sum  Inputs=-+
  Switch : Switch  Criteria=u2 > Threshold
  Transport Delay : TransportDelay  DelayTime=20000000  InitialOutput=1
  FLOW FRACTION : Outport
  HEAT TRANSFER FRACTION : Outport  Port=2
  wires:
  Transport Delay/1 -> 1-D Lookup Table/1, Scope/1, FLOW FRACTION/1
  Clock/1 -> Fcn/1
  Switch/1 -> Transport Delay/1
  Fcn/1 -> Subtract/1, Switch/1
  Final convection flow rate/1 -> Subtract/2, Switch/3
  Subtract/1 -> Switch/2
  1-D Lookup Table/1 -> HEAT TRANSFER FRACTION/1

== system MSDR_and_BOP_v1_1/HEAT EXCHANGERS/HEAT EXCHANGER LOOP 4/SHX1 HEAT TRANSFER ==
  PRIMARY FLUID INLET TEMPERATURE : Inport
  SECONDARY FLUID INLET TEMPERATURE : Inport  Port=2
  PRIMARY FLOW FRACTION : Inport  Port=3
  PRIMARY HEAT TRANSFER FRACTION : Inport  Port=4
  SECONDARY FLOW FRACTION : Inport  Port=5
  SECONDARY HEAT TRANSFER FRACTION : Inport  Port=6
  Mux : Mux  Inputs=16
      settings: DisplayOption=signals
  To Workspace : ToWorkspace  VariableName=shx1_ht  SampleTime=-1
  Tp1_shx1 : Integrator  InitialCondition=T0_p_shx1(1)
  Tp2_shx1 : Integrator  InitialCondition=T0_p_shx1(2)
  "Tp3_shx1 " : Integrator  InitialCondition=T0_p_shx1(3)
  Tp4_shx1 : Integrator  InitialCondition=T0_p_shx1(4)
  Ts1_shx1 : Integrator  InitialCondition=T0_s_shx1(1)
  Ts2_shx1 : Integrator  InitialCondition=T0_s_shx1(2)
  Ts3_shx1 : Integrator  InitialCondition=T0_s_shx1(3)
  Ts4_shx1 : Integrator  InitialCondition=T0_s_shx1(4)
  Tt1_shx1 : Integrator  InitialCondition=T0_t_shx1(1)
  Tt2_shx1 : Integrator  InitialCondition=T0_t_shx1(2)
  d(Tp1_shx1)/dt : Fcn  Expr=(u[13]*Wp_shx1/mp_shx1(1))*(u[1] - u[3]) + (u[14]*hA_p_shx1(1)/mcp_p_shx1(1))*(u[7] - u[3])
  d(Tp2_shx1)/dt : Fcn  Expr=(u[13]*Wp_shx1/mp_shx1(2))*(u[3] - u[4]) + (u[14]*hA_p_shx1(2)/mcp_p_shx1(2))*(u[7] - u[3])
  d(Tp3_shx1)/dt : Fcn  Expr=(u[13]*Wp_shx1/mp_shx1(3))*(u[4] - u[5]) + (u[14]*hA_p_shx1(3)/mcp_p_shx1(3))*(u[8] - u[5])
  d(Tp4_shx1)/dt : Fcn  Expr=(u[13]*Wp_shx1/mp_shx1(4))*(u[5] - u[6]) + (u[14]*hA_p_shx1(4)/mcp_p_shx1(4))*(u[8] - u[5])
  d(Ts1_shx1)/dt : Fcn  Expr=(u[15]*Ws_shx1/ms_shx1(1))*(u[2] - u[9]) + (u[16]*hA_s_shx1(1)/mcp_s_shx1(1))*(u[8] - u[9])
  d(Ts2_shx1)/dt : Fcn  Expr=(u[15]*Ws_shx1/ms_shx1(2))*(u[9] - u[10]) + (u[16]*hA_s_shx1(2)/mcp_s_shx1(2))*(u[8] - u[9])
  d(Ts3_shx1)/dt : Fcn  Expr=(u[15]*Ws_shx1/ms_shx1(3))*(u[10] - u[11]) + (u[16]*hA_s_shx1(3)/mcp_s_shx1(3))*(u[7] - u[11])
  d(Ts4_shx1)/dt : Fcn  Expr=(u[15]*Ws_shx1/ms_shx1(4))*(u[11] - u[12]) + (u[16]*hA_s_shx1(4)/mcp_s_shx1(4))*(u[7] - u[11])
  d(Tt1_shx1)/dt : Fcn  Expr=(u[14]*(hA_p_shx1(1) + hA_p_shx1(2))/mcp_t_shx1(1))*(u[3] - u[7]) + (u[16]*(hA_s_shx1(1) + hA_s_shx1(2))/mcp_t_shx1(1))*(u[11] - u[7])
  d(Tt2_shx1)/dt : Fcn  Expr=(u[14]*(hA_p_shx1(3) + hA_p_shx1(4))/mcp_t_shx1(2))*(u[5] - u[8]) + (u[16]*(hA_s_shx1(3) + hA_s_shx1(4))/mcp_t_shx1(2))*(u[9] - u[8])
  SHX1 TEMPERATURES : Outport
  wires:
  Ts1_shx1/1 -> Mux/9
  Ts2_shx1/1 -> Mux/10
  d(Ts2_shx1)/dt/1 -> Ts2_shx1/1
  d(Tp4_shx1)/dt/1 -> Tp4_shx1/1
  Tt1_shx1/1 -> Mux/7
  d(Tp2_shx1)/dt/1 -> Tp2_shx1/1
  Tp4_shx1/1 -> Mux/6
  d(Tt2_shx1)/dt/1 -> Tt2_shx1/1
  SECONDARY FLUID INLET TEMPERATURE/1 -> Mux/2
  Tt2_shx1/1 -> Mux/8
  Mux/1 -> To Workspace/1, SHX1 TEMPERATURES/1, d(Ts4_shx1)/dt/1, d(Ts3_shx1)/dt/1, d(Ts2_shx1)/dt/1, d(Ts1_shx1)/dt/1, d(Tt2_shx1)/dt/1, d(Tt1_shx1)/dt/1, d(Tp4_shx1)/dt/1, d(Tp3_shx1)/dt/1, d(Tp2_shx1)/dt/1, d(Tp1_shx1)/dt/1
  d(Tp1_shx1)/dt/1 -> Tp1_shx1/1
  d(Ts4_shx1)/dt/1 -> Ts4_shx1/1
  Tp1_shx1/1 -> Mux/3
  d(Ts1_shx1)/dt/1 -> Ts1_shx1/1
  d(Ts3_shx1)/dt/1 -> Ts3_shx1/1
  Ts3_shx1/1 -> Mux/11
  Ts4_shx1/1 -> Mux/12
  "Tp3_shx1 "/1 -> Mux/5
  d(Tp3_shx1)/dt/1 -> "Tp3_shx1 "/1
  Tp2_shx1/1 -> Mux/4
  d(Tt1_shx1)/dt/1 -> Tt1_shx1/1
  PRIMARY FLUID INLET TEMPERATURE/1 -> Mux/1
  PRIMARY HEAT TRANSFER FRACTION/1 -> Mux/14
  SECONDARY HEAT TRANSFER FRACTION/1 -> Mux/16
  PRIMARY FLOW FRACTION/1 -> Mux/13
  SECONDARY FLOW FRACTION/1 -> Mux/15

== system MSDR_and_BOP_v1_1/HEAT EXCHANGERS/HEAT EXCHANGER LOOP 4/SHX1 MATERIAL TRANSPORT ==
  SHX1 TEMPERATURES : Inport
  wires:
  SHX1 TEMPERATURES/1 -> ?

== system MSDR_and_BOP_v1_1/HEAT EXCHANGERS/HEAT EXCHANGER LOOP 4/SHX2 HEAT TRANSFER ==
  PRIMARY FLUID INLET TEMPERATURE : Inport
  SECONDARY FLUID INLET TEMPERATURE : Inport  Port=2
  PRIMARY FLOW FRACTION : Inport  Port=3
  PRIMARY HEAT TRANSFER FRACTION : Inport  Port=4
  SECONDARY FLOW FRACTION : Inport  Port=5
  SECONDARY HEAT TRANSFER FRACTION : Inport  Port=6
  Mux : Mux  Inputs=16
      settings: DisplayOption=signals
  To Workspace : ToWorkspace  VariableName=shx2_ht  SampleTime=-1
  Tp1_shx2 : Integrator  InitialCondition=T0_p_shx2(1)
  Tp2_shx2 : Integrator  InitialCondition=T0_p_shx2(2)
  "Tp3_shx2 " : Integrator  InitialCondition=T0_p_shx2(3)
  Tp4_shx2 : Integrator  InitialCondition=T0_p_shx2(4)
  Ts1_shx2 : Integrator  InitialCondition=T0_s_shx2(1)
  Ts2_shx2 : Integrator  InitialCondition=T0_s_shx2(2)
  Ts3_shx2 : Integrator  InitialCondition=T0_s_shx2(3)
  Ts4_shx2 : Integrator  InitialCondition=T0_s_shx2(4)
  Tt1_shx2 : Integrator  InitialCondition=T0_t_shx2(1)
  Tt2_shx2 : Integrator  InitialCondition=T0_t_shx2(2)
  d(Tp1_shx2)/dt : Fcn  Expr=(u[13]*Wp_shx2/mp_shx2(1))*(u[1] - u[3]) + (u[14]*hA_p_shx2(1)/mcp_p_shx2(1))*(u[7] - u[3])
  d(Tp2_shx2)/dt : Fcn  Expr=(u[13]*Wp_shx2/mp_shx2(2))*(u[3] - u[4]) + (u[14]*hA_p_shx2(2)/mcp_p_shx2(2))*(u[7] - u[3])
  d(Tp3_shx2)/dt : Fcn  Expr=(u[13]*Wp_shx2/mp_shx2(3))*(u[4] - u[5]) + (u[14]*hA_p_shx2(3)/mcp_p_shx2(3))*(u[8] - u[5])
  d(Tp4_shx2)/dt : Fcn  Expr=(u[13]*Wp_shx2/mp_shx2(4))*(u[5] - u[6]) + (u[14]*hA_p_shx2(4)/mcp_p_shx2(4))*(u[8] - u[5])
  d(Ts1_shx2)/dt : Fcn  Expr=(u[15]*Ws_shx2/ms_shx2(1))*(u[2] - u[9]) + (u[16]*hA_s_shx2(1)/mcp_s_shx2(1))*(u[8] - u[9])
  d(Ts2_shx2)/dt : Fcn  Expr=(u[15]*Ws_shx2/ms_shx2(2))*(u[9] - u[10]) + (u[16]*hA_s_shx2(2)/mcp_s_shx2(2))*(u[8] - u[9])
  d(Ts3_shx2)/dt : Fcn  Expr=(u[15]*Ws_shx2/ms_shx2(3))*(u[10] - u[11]) + (u[16]*hA_s_shx2(3)/mcp_s_shx2(3))*(u[7] - u[11])
  d(Ts4_shx2)/dt : Fcn  Expr=(u[15]*Ws_shx2/ms_shx2(4))*(u[11] - u[12]) + (u[16]*hA_s_shx2(4)/mcp_s_shx2(4))*(u[7] - u[11])
  d(Tt1_shx2)/dt : Fcn  Expr=(u[14]*(hA_p_shx2(1) + hA_p_shx2(2))/mcp_t_shx2(1))*(u[3] - u[7]) + (u[16]*(hA_s_shx2(1) + hA_s_shx2(2))/mcp_t_shx2(1))*(u[11] - u[7])
  d(Tt2_shx2)/dt : Fcn  Expr=(u[14]*(hA_p_shx2(3) + hA_p_shx2(4))/mcp_t_shx2(2))*(u[5] - u[8]) + (u[16]*(hA_s_shx2(3) + hA_s_shx2(4))/mcp_t_shx2(2))*(u[9] - u[8])
  SHX2 TEMPERATURES : Outport
  wires:
  Ts1_shx2/1 -> Mux/9
  Ts2_shx2/1 -> Mux/10
  d(Ts2_shx2)/dt/1 -> Ts2_shx2/1
  d(Tp4_shx2)/dt/1 -> Tp4_shx2/1
  Tt1_shx2/1 -> Mux/7
  d(Tp2_shx2)/dt/1 -> Tp2_shx2/1
  Tp4_shx2/1 -> Mux/6
  d(Tt2_shx2)/dt/1 -> Tt2_shx2/1
  SECONDARY FLUID INLET TEMPERATURE/1 -> Mux/2
  Tt2_shx2/1 -> Mux/8
  Mux/1 -> To Workspace/1, SHX2 TEMPERATURES/1, d(Ts4_shx2)/dt/1, d(Ts3_shx2)/dt/1, d(Ts2_shx2)/dt/1, d(Ts1_shx2)/dt/1, d(Tt2_shx2)/dt/1, d(Tt1_shx2)/dt/1, d(Tp4_shx2)/dt/1, d(Tp3_shx2)/dt/1, d(Tp2_shx2)/dt/1, d(Tp1_shx2)/dt/1
  d(Tp1_shx2)/dt/1 -> Tp1_shx2/1
  d(Ts4_shx2)/dt/1 -> Ts4_shx2/1
  Tp1_shx2/1 -> Mux/3
  d(Ts1_shx2)/dt/1 -> Ts1_shx2/1
  d(Ts3_shx2)/dt/1 -> Ts3_shx2/1
  Ts3_shx2/1 -> Mux/11
  Ts4_shx2/1 -> Mux/12
  "Tp3_shx2 "/1 -> Mux/5
  d(Tp3_shx2)/dt/1 -> "Tp3_shx2 "/1
  Tp2_shx2/1 -> Mux/4
  d(Tt1_shx2)/dt/1 -> Tt1_shx2/1
  PRIMARY FLUID INLET TEMPERATURE/1 -> Mux/1
  PRIMARY HEAT TRANSFER FRACTION/1 -> Mux/14
  SECONDARY FLOW FRACTION/1 -> Mux/15
  SECONDARY HEAT TRANSFER FRACTION/1 -> Mux/16
  PRIMARY FLOW FRACTION/1 -> Mux/13

== system MSDR_and_BOP_v1_1/HEAT EXCHANGERS/HEAT EXCHANGER LOOP 4/SHX2 MATERIAL TRANSPORT ==
  SHX2 TEMPERATURES : Inport
  wires:
  SHX2 TEMPERATURES/1 -> ?

== system MSDR_and_BOP_v1_1/HEAT EXCHANGERS/HEAT EXCHANGER LOOP 4/THX1 HEAT TRANSFER ==
  PRIMARY FLUID INLET TEMPERATURE : Inport
  SECONDARY FLUID INLET TEMPERATURE : Inport  Port=2
  PRIMARY FLOW FRACTION : Inport  Port=3
  PRIMARY HEAT TRANSFER FRACTION : Inport  Port=4
  SECONDARY FLOW FRACTION : Inport  Port=5
  SECONDARY HEAT TRANSFER FRACTION : Inport  Port=6
  Mux : Mux  Inputs=16
      settings: DisplayOption=signals
  To Workspace : ToWorkspace  VariableName=thx1_ht  SampleTime=-1
  Tp1_thx1 : Integrator  InitialCondition=T0_p_thx1(1)
  Tp2_thx1 : Integrator  InitialCondition=T0_p_thx1(2)
  "Tp3_thx1 " : Integrator  InitialCondition=T0_p_thx1(3)
  Tp4_thx1 : Integrator  InitialCondition=T0_p_thx1(4)
  Ts1_thx1 : Integrator  InitialCondition=T0_s_thx1(1)
  Ts2_thx1 : Integrator  InitialCondition=T0_s_thx1(2)
  Ts3_thx1 : Integrator  InitialCondition=T0_s_thx1(3)
  Ts4_thx1 : Integrator  InitialCondition=T0_s_thx1(4)
  Tt1_thx1 : Integrator  InitialCondition=T0_t_thx1(1)
  Tt2_thx1 : Integrator  InitialCondition=T0_t_thx1(2)
  d(Tp1_thx1)/dt : Fcn  Expr=(u[13]*Wp_thx1/mp_thx1(1))*(u[1] - u[3]) + (u[14]*hA_p_thx1(1)/mcp_p_thx1(1))*(u[7] - u[3])
  d(Tp2_thx1)/dt : Fcn  Expr=(u[13]*Wp_thx1/mp_thx1(2))*(u[3] - u[4]) + (u[14]*hA_p_thx1(2)/mcp_p_thx1(2))*(u[7] - u[3])
  d(Tp3_thx1)/dt : Fcn  Expr=(u[13]*Wp_thx1/mp_thx1(3))*(u[4] - u[5]) + (u[14]*hA_p_thx1(3)/mcp_p_thx1(3))*(u[8] - u[5])
  d(Tp4_thx1)/dt : Fcn  Expr=(u[13]*Wp_thx1/mp_thx1(4))*(u[5] - u[6]) + (u[14]*hA_p_thx1(4)/mcp_p_thx1(4))*(u[8] - u[5])
  d(Ts1_thx1)/dt : Fcn  Expr=(u[15]*Ws_thx1/ms_thx1(1))*(u[2] - u[9]) + (u[16]*hA_s_thx1(1)/mcp_s_thx1(1))*(u[8] - u[9])
  d(Ts2_thx1)/dt : Fcn  Expr=(u[15]*Ws_thx1/ms_thx1(2))*(u[9] - u[10]) + (u[16]*hA_s_thx1(2)/mcp_s_thx1(2))*(u[8] - u[9])
  d(Ts3_thx1)/dt : Fcn  Expr=(u[15]*Ws_thx1/ms_thx1(3))*(u[10] - u[11]) + (u[16]*hA_s_thx1(3)/mcp_s_thx1(3))*(u[7] - u[11])
  d(Ts4_thx1)/dt : Fcn  Expr=(u[15]*Ws_thx1/ms_thx1(4))*(u[11] - u[12]) + (u[16]*hA_s_thx1(4)/mcp_s_thx1(4))*(u[7] - u[11])
  d(Tt1_thx1)/dt : Fcn  Expr=(u[14]*(hA_p_thx1(1) + hA_p_thx1(2))/mcp_t_thx1(1))*(u[3] - u[7]) + (u[16]*(hA_s_thx1(1) + hA_s_thx1(2))/mcp_t_thx1(1))*(u[11] - u[7])
  d(Tt2_thx1)/dt : Fcn  Expr=(u[14]*(hA_p_thx1(3) + hA_p_thx1(4))/mcp_t_thx1(2))*(u[5] - u[8]) + (u[16]*(hA_s_thx1(3) + hA_s_thx1(4))/mcp_t_thx1(2))*(u[9] - u[8])
  THX TEMPERATURES : Outport
  wires:
  Ts1_thx1/1 -> Mux/9
  Ts2_thx1/1 -> Mux/10
  d(Ts2_thx1)/dt/1 -> Ts2_thx1/1
  d(Tp4_thx1)/dt/1 -> Tp4_thx1/1
  Tt1_thx1/1 -> Mux/7
  d(Tp2_thx1)/dt/1 -> Tp2_thx1/1
  Tp4_thx1/1 -> Mux/6
  d(Tt2_thx1)/dt/1 -> Tt2_thx1/1
  SECONDARY FLUID INLET TEMPERATURE/1 -> Mux/2
  Tt2_thx1/1 -> Mux/8
  Mux/1 -> To Workspace/1, THX TEMPERATURES/1, d(Ts4_thx1)/dt/1, d(Ts3_thx1)/dt/1, d(Ts2_thx1)/dt/1, d(Ts1_thx1)/dt/1, d(Tt2_thx1)/dt/1, d(Tt1_thx1)/dt/1, d(Tp4_thx1)/dt/1, d(Tp3_thx1)/dt/1, d(Tp2_thx1)/dt/1, d(Tp1_thx1)/dt/1
  d(Tp1_thx1)/dt/1 -> Tp1_thx1/1
  d(Ts4_thx1)/dt/1 -> Ts4_thx1/1
  Tp1_thx1/1 -> Mux/3
  d(Ts1_thx1)/dt/1 -> Ts1_thx1/1
  d(Ts3_thx1)/dt/1 -> Ts3_thx1/1
  Ts3_thx1/1 -> Mux/11
  Ts4_thx1/1 -> Mux/12
  "Tp3_thx1 "/1 -> Mux/5
  d(Tp3_thx1)/dt/1 -> "Tp3_thx1 "/1
  Tp2_thx1/1 -> Mux/4
  d(Tt1_thx1)/dt/1 -> Tt1_thx1/1
  PRIMARY FLUID INLET TEMPERATURE/1 -> Mux/1
  PRIMARY FLOW FRACTION/1 -> Mux/13
  PRIMARY HEAT TRANSFER FRACTION/1 -> Mux/14
  SECONDARY FLOW FRACTION/1 -> Mux/15
  SECONDARY HEAT TRANSFER FRACTION/1 -> Mux/16

== system MSDR_and_BOP_v1_1/HEAT EXCHANGERS/HEAT EXCHANGER LOOP 4/THX1 MATERIAL TRANSPORT ==
  THX TEMPERATURES : Inport
  wires:
  THX TEMPERATURES/1 -> ?

== system MSDR_and_BOP_v1_1/HEAT EXCHANGERS/HEAT EXCHANGER LOOP 5/BOILER & REHEATER ==
  Coolant Inlet Temp : Inport
  Power Demand (Frac) : Inport  Port=2
  Fcn : Fcn  Commented=on  Expr=u[1] - u[2]*250/((Ws_shx1 + Ws_shx2)*Cp_s_shx)
  Integrator : Integrator  InitialCondition=400
  Mux : Mux  Inputs=3
      settings: DisplayOption=signals
  To Workspace : ToWorkspace  VariableName=msdr_br_mux2  SampleTime=-1
  ddt_t_b = 1/tau_b*(t_bin-t_b)-p_b/mb_cpb : Fcn  Expr=W_sb*(u(1)-u(3))/m_sb - u(2)/mb_cpb
  Coolant Exit Temp : Outport
  wires:
  Integrator/1 -> Coolant Exit Temp/1, Mux/3
  Mux/1 -> ddt_t_b = 1/tau_b*(t_bin-t_b)-p_b/mb_cpb/1, To Workspace/1
  Power Demand (Frac)/1 -> Mux/2
  Coolant Inlet Temp/1 -> Mux/1
  ddt_t_b = 1/tau_b*(t_bin-t_b)-p_b/mb_cpb/1 -> Integrator/1

== system MSDR_and_BOP_v1_1/HEAT EXCHANGERS/HEAT EXCHANGER LOOP 5/Fractional Power Demand (fractional) ==
  Add : Sum
  Constant : Constant
  Saturation : Saturate  UpperLimit=1  LowerLimit=0.2
  Saturation1 : Saturate  UpperLimit=.8  LowerLimit=0
  Slider : SliderBlock
  down 1%/min : simulink/Sources/Ramp  slope=-0.01/60  start=2500  InitialOutput=1
  up 1%/min1 : simulink/Sources/Ramp  slope=0.01/60  start=2500+3600+5000  InitialOutput=0
  Power Demand(frac) : Outport
  wires:
  down 1%/min/1 -> Saturation/1
  Saturation/1 -> Add/1
  up 1%/min1/1 -> Saturation1/1
  Saturation1/1 -> Add/2
  Constant/1 -> Power Demand(frac)/1

== system MSDR_and_BOP_v1_1/HEAT EXCHANGERS/HEAT EXCHANGER LOOP 5/PHX PRIM MIXING ==
  Tp_phx3 : Inport
  Tp_phx4 : Inport  Port=2
  p_flow_frac : Inport  Port=3
  Fcn : Fcn  Expr=u[3]*Wp_phx3/mp_phxm*(u[1]-u[4]) + u[3]*Wp_phx4/mp_phxm*(u[2]-u[4])
  Integrator : Integrator  InitialCondition=Tf_in
  Mux : Mux
  Tp_phx_mix : Outport
  wires:
  Tp_phx3/1 -> Mux/1
  Tp_phx4/1 -> Mux/2
  Mux/1 -> Fcn/1
  p_flow_frac/1 -> Mux/3
  Fcn/1 -> Integrator/1
  Integrator/1 -> Tp_phx_mix/1, Mux/4

== system MSDR_and_BOP_v1_1/HEAT EXCHANGERS/HEAT EXCHANGER LOOP 5/PHX SEC MIXING ==
  Ts_phx3 : Inport
  Ts_phx4 : Inport  Port=2
  s_flow_frac : Inport  Port=3
  Fcn : Fcn  Expr=u[3]*Ws_phx3/ms_phxm*(u[1]-u[4]) + u[3]*Ws_phx4/ms_phxm*(u[2]-u[4])
  Integrator : Integrator  InitialCondition=T0_s_phx1(4)
  Mux : Mux
  Ts_phx_mix : Outport
  wires:
  Ts_phx3/1 -> Mux/1
  Ts_phx4/1 -> Mux/2
  Mux/1 -> Fcn/1
  s_flow_frac/1 -> Mux/3
  Fcn/1 -> Integrator/1
  Integrator/1 -> Ts_phx_mix/1, Mux/4

== system MSDR_and_BOP_v1_1/HEAT EXCHANGERS/HEAT EXCHANGER LOOP 5/PHX//SHX PUMP ==
  1-D Lookup Table : Lookup_n-D  NumberOfTableDimensions=1  BreakpointsForDimension1=xdat  Table=ydat  InternalRulePriority=Speed  RndMeth=Simplest  InputSameDT=on
  Clock : Clock
  Fcn : Fcn  Expr=exp((1/tau_p)*u)
  Final convection flow rate : Constant  Value=therm_conv
  Scope : Scope
  Subtract : Sum  Inputs=-+
  Switch : Switch  Criteria=u2 > Threshold
  Transport Delay : TransportDelay  DelayTime=60000000  InitialOutput=1
  FLOW FRACTION : Outport
  HEAT TRANSFER FRACTION : Outport  Port=2
  wires:
  Transport Delay/1 -> 1-D Lookup Table/1, Scope/1, FLOW FRACTION/1
  Clock/1 -> Fcn/1
  Switch/1 -> Transport Delay/1
  Fcn/1 -> Subtract/1, Switch/1
  Final convection flow rate/1 -> Subtract/2, Switch/3
  Subtract/1 -> Switch/2
  1-D Lookup Table/1 -> HEAT TRANSFER FRACTION/1
